simulink library "misc_lib"  (R2017b)
settings: Solver=VariableStepAuto  StartTime=0.0  StopTime=10.0  RelTol=1e-3
values from neighbouring files (symbols this model uses):
  L1 = Lsl + Lm    (= 0.098)    [control_params.m]
  Lm = 92.6e-3    (= 0.0926)    [control_params.m]
  Lrl = 4.9e-3    (= 0.0049)    [control_params.m]
  sw_table = [ra; rb; rc; rd; re; rf]    [switching_table_params.m]
  Tr = L2/R2    (= 0.0691489361702)    [control_params.m]
  Tsamp = 0.0001    [control_params.m]
  Udc = 60    [control_params.m]
undefined symbols (not defined in the file or in its folder): DiscIntNeverNeededParam
libraries: coordinate_transform_lib x2
settings Model: Creator=Máté  LastModifiedBy=Máté

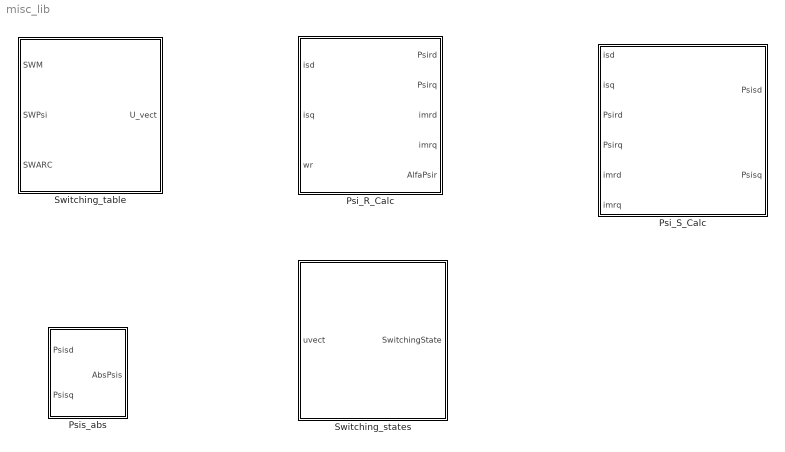
== system misc_lib ==
  Psi_R_Calc : Subsystem
  Psi_S_Calc : Subsystem
  Psis_abs : Subsystem
  "Switching_states " : Subsystem
  Switching_table : Subsystem

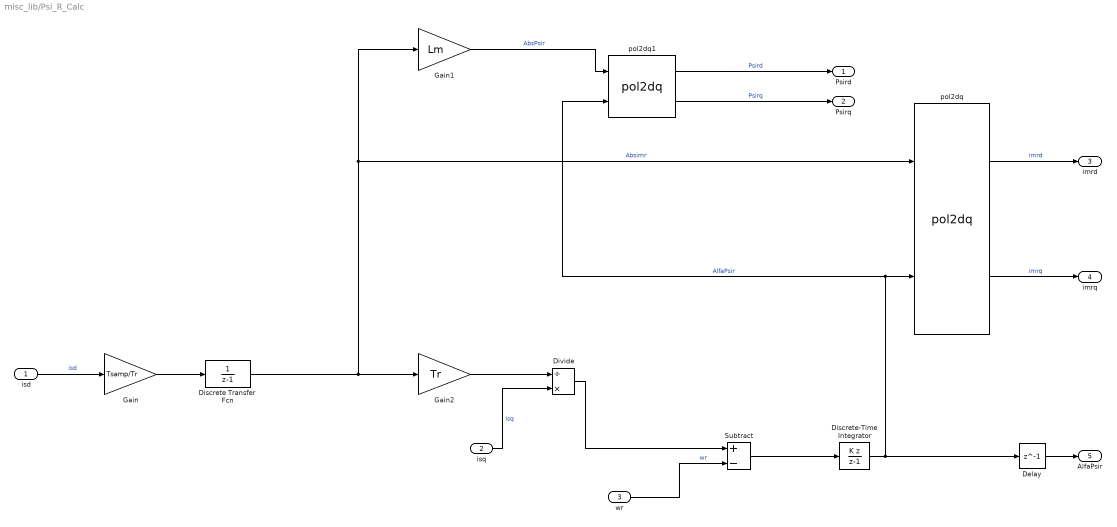
== system misc_lib/Psi_R_Calc ==
  isd : Inport
  isq : Inport  Port=2
  wr : Inport  Port=3
  Delay : Delay  DelayLength=1
  Discrete Transfer Fcn : DiscreteTransferFcn  Denominator=[1 -1]
  Discrete-Time Integrator : DiscreteIntegrator  IntegratorMethod=Accumulation: Backward Euler  InitialConditionSetting=State (most efficient)  SampleTime=-1  ICPrevOutput=DiscIntNeverNeededParam  ICPrevScaledInput=DiscIntNeverNeededParam
  Divide : Product  Inputs=/*
  Gain : Gain  Gain=Tsamp/Tr
  Gain1 : Gain  Gain=Lm
  Gain2 : Gain  Gain=Tr
  Subtract : Sum  Inputs=+-
  pol2dq : coordinate_transform_lib/pol2dq
  pol2dq1 : coordinate_transform_lib/pol2dq
  Psird : Outport
  Psirq : Outport  Port=2
  imrd : Outport  Port=3
  imrq : Outport  Port=4
  AlfaPsir : Outport  Port=5
  wires:
  Gain1/1 -> pol2dq1/1  "AbsPsir"
  wr/1 -> Subtract/2  "wr"
  isq/1 -> Divide/2  "isq"
  pol2dq/1 -> imrd/1  "imrd"
  Subtract/1 -> Discrete-Time Integrator/1
  Discrete-Time Integrator/1 -> Delay/1, pol2dq/2, pol2dq1/2  "AlfaPsir"
  Gain/1 -> Discrete Transfer Fcn/1
  Gain2/1 -> Divide/1
  Divide/1 -> Subtract/1
  isd/1 -> Gain/1  "isd"
  Discrete Transfer Fcn/1 -> Gain1/1, pol2dq/1, Gain2/1  "Absimr"
  pol2dq/2 -> imrq/1  "imrq"
  pol2dq1/2 -> Psirq/1  "Psirq"
  pol2dq1/1 -> Psird/1  "Psird"
  Delay/1 -> AlfaPsir/1

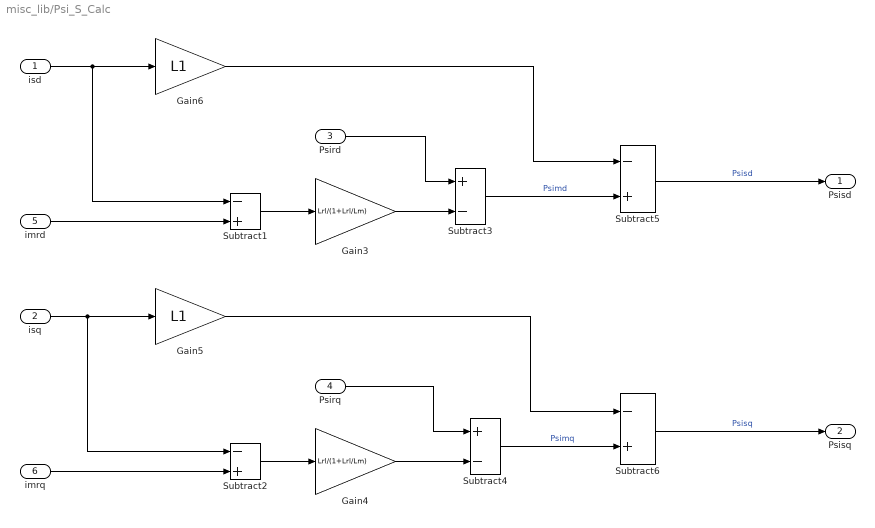
== system misc_lib/Psi_S_Calc ==
  isd : Inport
  isq : Inport  Port=2
  Psird : Inport  Port=3
  Psirq : Inport  Port=4
  imrd : Inport  Port=5
  imrq : Inport  Port=6
  Gain3 : Gain  Gain=Lrl/(1+Lrl/Lm)
  Gain4 : Gain  Gain=Lrl/(1+Lrl/Lm)
  Gain5 : Gain  Gain=L1
  Gain6 : Gain  Gain=L1
  Subtract{1..2,5..6} (4 alike) : Sum  Inputs=-+
  Subtract3 : Sum  Inputs=+-
  Subtract4 : Sum  Inputs=+-
  Psisd : Outport
  Psisq : Outport  Port=2
  wires:
  Gain5/1 -> Subtract6/1
  Gain4/1 -> Subtract4/2
  Subtract4/1 -> Subtract6/2  "Psimq"
  Gain3/1 -> Subtract3/2
  Subtract3/1 -> Subtract5/2  "Psimd"
  Subtract1/1 -> Gain3/1
  Subtract2/1 -> Gain4/1
  Gain6/1 -> Subtract5/1
  isq/1 -> Subtract2/1, Gain5/1
  isd/1 -> Subtract1/1, Gain6/1
  Subtract5/1 -> Psisd/1  "Psisd"
  Subtract6/1 -> Psisq/1  "Psisq"
  imrd/1 -> Subtract1/2
  imrq/1 -> Subtract2/2
  Psird/1 -> Subtract3/1
  Psirq/1 -> Subtract4/1

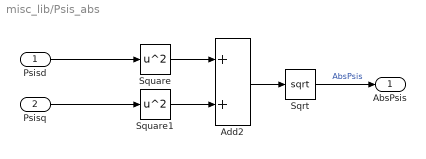
== system misc_lib/Psis_abs ==
  Psisd : Inport
  Psisq : Inport  Port=2
  Add2 : Sum
  Sqrt : Sqrt  SaturateOnIntegerOverflow=on
  Square : Math  Operator=square  RndMeth=Zero  SaturateOnIntegerOverflow=on
  Square1 : Math  Operator=square  RndMeth=Zero  SaturateOnIntegerOverflow=on
  AbsPsis : Outport
  wires:
  Sqrt/1 -> AbsPsis/1  "AbsPsis"
  Square1/1 -> Add2/2
  Square/1 -> Add2/1
  Add2/1 -> Sqrt/1
  Psisd/1 -> Square/1
  Psisq/1 -> Square1/1

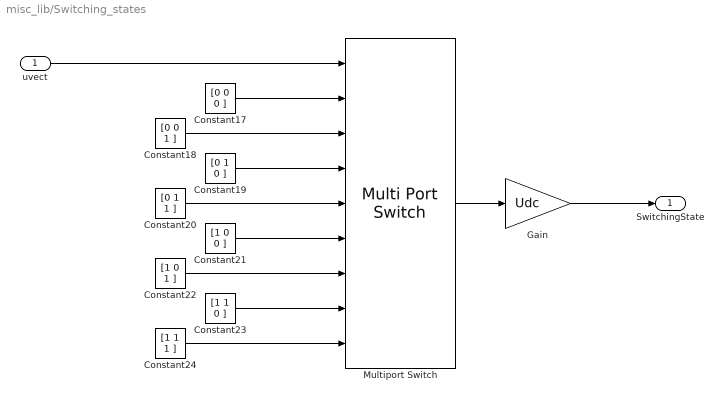
== system misc_lib/Switching_states  ==
  uvect : Inport
  Constant17 : Constant  Value=[0 0 0 ]
  Constant18 : Constant  Value=[0 0 1 ]
  Constant19 : Constant  Value=[0 1 0 ]
  Constant20 : Constant  Value=[0 1 1 ]
  Constant21 : Constant  Value=[1 0 0 ]
  Constant22 : Constant  Value=[1 0 1 ]
  Constant23 : Constant  Value=[1 1 0 ]
  Constant24 : Constant  Value=[1 1 1 ]
  Gain : Gain  Gain=Udc
  Multiport Switch : MultiPortSwitch  DataPortOrder=Zero-based contiguous  Inputs=8
  SwitchingState : Outport
  wires:
  Constant21/1 -> Multiport Switch/6
  Constant19/1 -> Multiport Switch/4
  uvect/1 -> Multiport Switch/1
  Constant17/1 -> Multiport Switch/2
  Constant18/1 -> Multiport Switch/3
  Constant24/1 -> Multiport Switch/9
  Gain/1 -> SwitchingState/1
  Constant23/1 -> Multiport Switch/8
  Constant22/1 -> Multiport Switch/7
  Multiport Switch/1 -> Gain/1
  Constant20/1 -> Multiport Switch/5

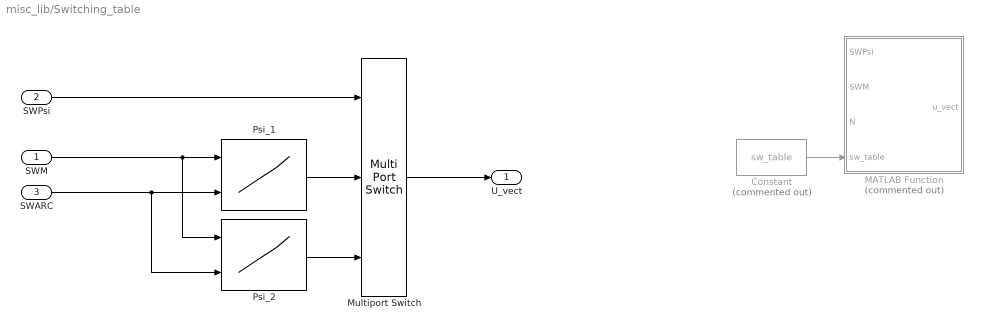
== system misc_lib/Switching_table ==
  SWM : Inport
  SWPsi : Inport  Port=2
  SWARC : Inport  Port=3
  Constant : Constant  Commented=on  Value=sw_table
  MATLAB Function : MATLAB Function  Commented=on  TreatAsAtomicUnit=on
  Multiport Switch : MultiPortSwitch  Inputs=2
  Psi_1 : Lookup2D  RowIndex=[1;2;3]  ColumnIndex=[1;2;3;4;5;6]  Table=[2 3 4 5 6 1;0 7 0 7 0 7;6 1 2 3 4 5]  SaturateOnIntegerOverflow=on
  Psi_2 : Lookup2D  RowIndex=[1;2;3]  ColumnIndex=[1;2;3;4;5;6]  Table=[3 4 5 6 1 2;7 0 7 0 7 0;5 6 1 2 3 4]  SaturateOnIntegerOverflow=on
  U_vect : Outport
  wires:
  Constant/1 -> MATLAB Function/4(sw_table)
  SWPsi/1 -> Multiport Switch/1
  Psi_2/1 -> Multiport Switch/3
  Psi_1/1 -> Multiport Switch/2
  SWM/1 -> Psi_2/1, Psi_1/1
  SWARC/1 -> Psi_2/2, Psi_1/2
  Multiport Switch/1 -> U_vect/1

== matlab function misc_lib/Switching_table/MATLAB Function ==
  data: SWPsi input; u_vect output; SWM input; N input; sw_table input
function u_vect = switching_function(SWPsi, SWM, N, sw_table)

double temp;

if (SWPsi == 1) && (SWM == 1)
    temp = sw_table(1,N);
    elseif (SWPsi == 1) && (SWM == 0)
        temp = sw_table(2,N);
        elseif (SWPsi == 1) && (SWM == -1)
            temp = sw_table(3,N);
            elseif (SWPsi == 0) && (SWM == 1)
                temp = sw_table(4,N);
                elseif (SWPsi == 0) && (SWM == 0)
                    temp = sw_table(5,N);
else 
    temp = sw_table(6,N);
end  

u_vect = temp;
